simulink model "base_model"  (R2022b)
settings: Solver=FixedStepAuto  StartTime=0.0  StopTime=inf  FixedStep=0.01  RelTol=1e-3
undefined symbols (not defined in the file or in its folder): National_Instruments, PCIe
libraries: sldrtlib x2
settings Model: SimulationMode=external  Creator=Fox I (Daniel)  LastModifiedBy=Group 1
settings SolverCC: AlgebraicLoopSolver=TrustRegion
settings DataIOCC: ReturnWorkspaceOutputs=off
settings DebuggingCC: UnconnectedInputMsg=warning  UnconnectedOutputMsg=warning  UnconnectedLineMsg=warning  SFMachineParentedDataDiag=warning  ArithmeticOperatorsInVariantConditions=warning
settings HardwareCC: ProdBitPerLong=64  ProdHWDeviceType=Intel->x86-64 (Linux 64)
settings ModelReferenceCC: EnableRefExpFcnMdlSchedulingChecks=on
settings SFSimCC: SimUseLocalCustomCode=off  CustomCodeUndefinedFunction=UseInterfaceOnly
settings RTWCC: Description=Simulink Desktop Real-Time  SystemTargetFile=sldrt.tlc  TemplateMakefile=sldrt.tmf  RTWUseLocalCustomCode=off  RTWCompilerOptimization=on  DLArmComputeVersion=19.05
settings CodeAppCC: MaxIdLength=95
settings SimulinkDesktopRealTimeCC: TargetLibSuffix=_sldrt.a  TargetPreCompLibLocation=C:\Program Files\MATLAB\R2022b\toolbox\sldrt\lib\win64

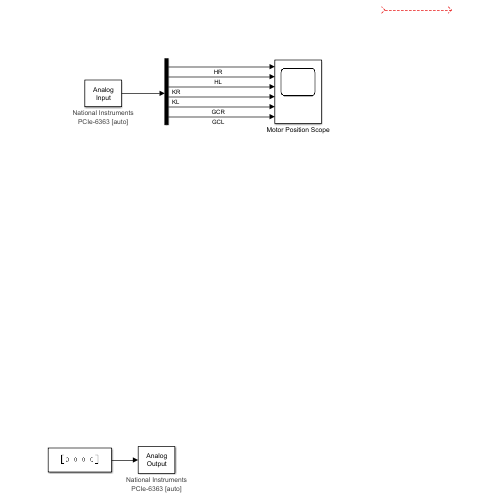
[thumbnail: Simulink's stored preview of the top-level diagram]
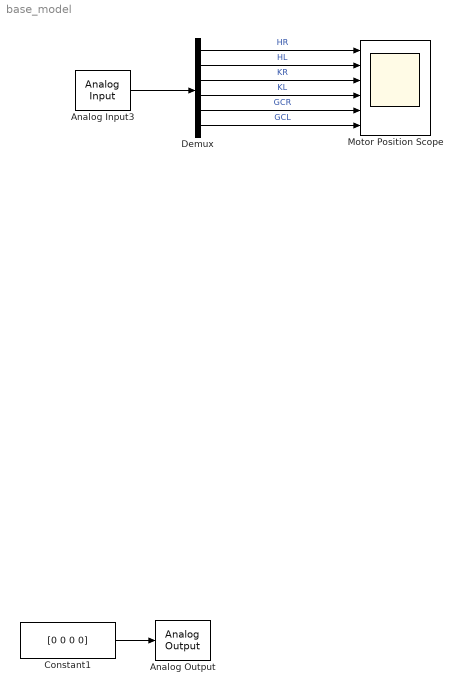
== system base_model ==
  Analog Input3 : sldrtlib/Analog Input  SampleTime=0.01  MaxMissedTicks=20  ShowMissedTicks=off  YieldWhenWaiting=off  DrvName=National_Instruments/PCIe-6363  DrvAddress=4294967295  DrvOptions=[0 0 0 0 0 0 0]  Channels=[1 2 3 4 5 6]  RangeMode=1  VoltRange=1  DataType=1
      settings: AttributesFormatString=National Instruments\nPCIe-6363 [auto]
  Analog Output : sldrtlib/Analog Output  SampleTime=0.01  MaxMissedTicks=100  ShowMissedTicks=off  YieldWhenWaiting=off  DrvName=National_Instruments/PCIe-6363  DrvAddress=4294967295  DrvOptions=[0 0 0 0 0 0 0]  Channels=[1 2 3 4]  RangeMode=1  VoltRange=1  InitialValue=0  FinalValue=0
      settings: AttributesFormatString=National Instruments\nPCIe-6363 [auto]
  Constant1 : Constant  Value=[0 0 0 0]
  Demux : Demux  Outputs=6
  Motor Position Scope : Scope  NumInputPorts=6
  wires:
  Analog Input3/1 -> Demux/1
  Demux/2 -> Motor Position Scope/2  "HL"
  Demux/1 -> Motor Position Scope/1  "HR"
  Demux/3 -> Motor Position Scope/3  "KR"
  Constant1/1 -> Analog Output/1
  ? -> ?
  Demux/4 -> Motor Position Scope/4  "KL"
  Demux/5 -> Motor Position Scope/5  "GCR"
  Demux/6 -> Motor Position Scope/6  "GCL"
